simulink model "foot_placement_controller_in_simulink"  (R2019a)
settings: Solver=ode5  StartTime=0.0  StopTime=180  FixedStep=.005  RelTol=1e-3  EnableMultiTasking=on
undefined symbols (not defined in the file): CAN_Device, National_Instruments, PCI, Vector
libraries: dsparch4 x10, sldrtlib x5
settings Model: SimulationMode=external  ExtModeTrigDuration=60001  Creator=SD55648  LastModifiedBy=Huawei Wang
settings DataIOCC: LimitDataPoints=on  SaveFormat=Array  ReturnWorkspaceOutputs=off
settings OptimizationCC: LifeSpan=inf
settings DebuggingCC: SolverPrmCheckMsg=warning  SFUnexpectedBacktrackingDiag=warning  SFNoUnconditionalDefaultTransitionDiag=warning  SFExecutionAtInitializationDiag=none  ArithmeticOperatorsInVariantConditions=warning
settings HardwareCC: TargetBitPerLong=64  TargetBitPerPointer=64  TargetIntDivRoundTo=Zero  TargetEndianess=LittleEndian  TargetWordSize=64  TargetHWDeviceType=Intel->x86-64
settings ModelReferenceCC: PropagateSignalLabelsOutOfModel=off
settings SFSimCC: SimUseLocalCustomCode=off
settings RTWCC: SystemTargetFile=sldrt.tlc  TemplateMakefile=sldrt.tmf  Description=Simulink Desktop Real-Time  RTWUseLocalCustomCode=off  RTWCompilerOptimization=on
settings CodeAppCC: MaxIdLength=95  StateflowObjectComments=on
settings SimulinkDesktopRealTimeCC: TargetPreCompLibLocation=C:\Program Files\MATLAB\R2019a\toolbox\sldrt\lib\win64  TargetLangStandard=C89/C90 (ANSI)  SupportVariableSizeSignals=off  PreserveStateflowLocalDataDimensions=off
settings ConfigComp: CovMetricSettings=dw  CovHtmlReporting=on  CovSaveCumulativeToWorkspaceVar=on  CovSaveSingleToWorkspaceVar=on  CovExternalEMLEnable=off  CovSFcnEnable=off

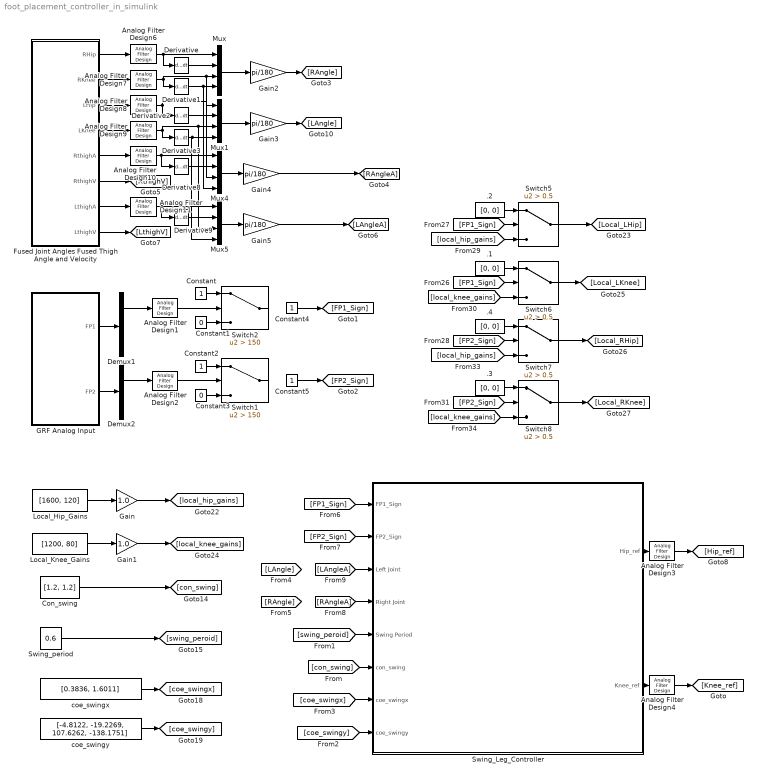
== system foot_placement_controller_in_simulink ==
  .{1..4} (4 alike) : Constant  Value=[0, 0]
  Analog Filter Design{1..4,6..11} (10 alike) : dsparch4/Analog Filter Design  method=Butterworth  filttype=Lowpass  N=2  Wlo=6*2*pi  Whi=80  Rp=2  Rs=40
  Con_swing : Constant  Value=[1.2, 1.2]
  Constant{,2,4..5} (4 alike) : Constant
  Constant1 : Constant  Value=0
  Constant3 : Constant  Value=0
  Demux1 : Demux  Outputs=6
  Demux2 : Demux  Outputs=6
  Derivative{,1..3,8..9} (6 alike) : Derivative
  Fused Joint Angles Fused Thigh Angle and Velocity : Subsystem
  "GRF Analog Input " : Subsystem
  Gain : Gain  Gain=1.0
  Gain1 : Gain  Gain=1.0
  Gain{2..5} (4 alike) : Gain  Gain=pi/180
  Local_Hip_Gains : Constant  Value=[1600, 120]
  Local_Knee_Gains : Constant  Value=[1200, 80]
  Mux{,1,4..5} (4 alike) : Mux
  "Swing_Leg_Controller " : Subsystem
  Swing_period : Constant  Value=0.6
  Switch1 : Switch  Criteria=u2 > Threshold  Threshold=150
  Switch2 : Switch  Criteria=u2 > Threshold  Threshold=150
  Switch{5..8} (4 alike) : Switch  Criteria=u2 > Threshold  Threshold=0.5
  coe_swingx : Constant  Value=[0.3836, 1.6011]
  coe_swingy : Constant  Value=[-4.8122, -19.2269, 107.6262, -138.1751]
  wires:
  Demux2/2 -> Analog Filter Design2/1
  "GRF Analog Input "/1(FP1) -> Demux1/1
  "GRF Analog Input "/2(FP2) -> Demux2/1
  Fused Joint Angles Fused Thigh Angle and Velocity/3(LHip) -> Analog Filter Design8/1
  Fused Joint Angles Fused Thigh Angle and Velocity/4(LKnee) -> Analog Filter Design9/1
  Fused Joint Angles Fused Thigh Angle and Velocity/5(RthighA) -> Analog Filter Design10/1
  Fused Joint Angles Fused Thigh Angle and Velocity/6(RthighV) -> [RthighV]
  Fused Joint Angles Fused Thigh Angle and Velocity/7(LthighA) -> Analog Filter Design11/1
  Fused Joint Angles Fused Thigh Angle and Velocity/8(LthighV) -> [LthighV]
  Derivative2/1 -> Mux1/2
  Derivative3/1 -> Mux1/4, Mux5/4
  Fused Joint Angles Fused Thigh Angle and Velocity/1(RHip) -> Analog Filter Design6/1
  Derivative/1 -> Mux/2
  Fused Joint Angles Fused Thigh Angle and Velocity/2(RKnee) -> Analog Filter Design7/1
  Derivative1/1 -> Mux4/4, Mux/4
  Mux1/1 -> Gain3/1
  Demux1/2 -> Analog Filter Design1/1
  Constant/1 -> Switch2/1
  Constant1/1 -> Switch2/3
  Constant2/1 -> Switch1/1
  Constant3/1 -> Switch1/3
  Mux/1 -> Gain2/1
  Gain3/1 -> [LAngle]
  Gain2/1 -> [RAngle]
  Con_swing/1 -> [con_swing]
  Swing_period/1 -> [swing_peroid]
  coe_swingx/1 -> [coe_swingx]
  [FP1_Sign] -> Switch5/2
  Local_Hip_Gains/1 -> Gain/1
  Local_Knee_Gains/1 -> Gain1/1
  [local_hip_gains] -> Switch5/3
  .2/1 -> Switch5/1
  [FP1_Sign] -> Switch6/2
  [local_knee_gains] -> Switch6/3
  .1/1 -> Switch6/1
  [FP2_Sign] -> Switch7/2
  [local_hip_gains] -> Switch7/3
  .4/1 -> Switch7/1
  [FP2_Sign] -> Switch8/2
  [local_knee_gains] -> Switch8/3
  .3/1 -> Switch8/1
  Switch5/1 -> [Local_LHip]
  Switch6/1 -> [Local_LKnee]
  Switch7/1 -> [Local_RHip]
  Switch8/1 -> [Local_RKnee]
  coe_swingy/1 -> [coe_swingy]
  [con_swing] -> "Swing_Leg_Controller "/6(con_swing)
  [swing_peroid] -> "Swing_Leg_Controller "/5(Swing Period)
  [coe_swingy] -> "Swing_Leg_Controller "/8(coe_swingy)
  [coe_swingx] -> "Swing_Leg_Controller "/7(coe_swingx)
  [LAngleA] -> "Swing_Leg_Controller "/3(Left Joint)
  [RAngleA] -> "Swing_Leg_Controller "/4(Right Joint)
  [FP1_Sign] -> "Swing_Leg_Controller "/1(FP1_Sign)
  [FP2_Sign] -> "Swing_Leg_Controller "/2(FP2_Sign)
  Gain/1 -> [local_hip_gains]
  Gain1/1 -> [local_knee_gains]
  Analog Filter Design6/1 -> Mux/1, Derivative/1
  Analog Filter Design7/1 -> Derivative1/1, Mux4/3, Mux/3
  Analog Filter Design8/1 -> Mux1/1, Derivative2/1
  Analog Filter Design9/1 -> Derivative3/1, Mux1/3, Mux5/3
  Analog Filter Design10/1 -> Mux4/1, Derivative8/1
  Analog Filter Design11/1 -> Derivative9/1, Mux5/1
  Derivative8/1 -> Mux4/2
  Mux4/1 -> Gain4/1
  Derivative9/1 -> Mux5/2
  Gain5/1 -> [LAngleA]
  Mux5/1 -> Gain5/1
  Gain4/1 -> [RAngleA]
  Analog Filter Design1/1 -> Switch2/2
  Analog Filter Design2/1 -> Switch1/2
  "Swing_Leg_Controller "/2(Knee_ref) -> Analog Filter Design4/1
  "Swing_Leg_Controller "/1("Hip_ref ") -> Analog Filter Design3/1
  Analog Filter Design3/1 -> [Hip_ref]
  Analog Filter Design4/1 -> [Knee_ref]
  Constant4/1 -> [FP1_Sign]
  Constant5/1 -> [FP2_Sign]

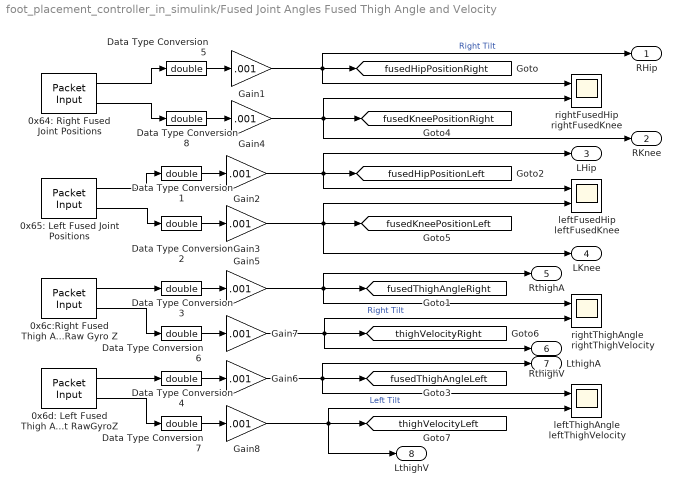
== system foot_placement_controller_in_simulink/Fused Joint Angles Fused Thigh Angle and Velocity ==
  0x64: Right Fused Joint Positions : sldrtlib/Packet Input  SampleTime=.005  MaxMissedTicks=10  ShowMissedTicks=off  YieldWhenWaiting=off  DrvName=Vector/CAN_Device  DrvAddress=1  DrvOptions=[0 0 0 0 1000]  PacketSize=8  DataTypes={'int32','int32'}  ShowReady=off  ShowError=off  PacketID=2048e0 + (hex2dec('64'))  ByteOrder=1  ShowTimestamp=off
      settings: AttributesFormatString=Vector\nCAN Device [1h]  SourceProductName=Simulink Desktop Real-Time
  0x65: Left Fused Joint Positions : sldrtlib/Packet Input  SampleTime=.005  MaxMissedTicks=10  ShowMissedTicks=off  YieldWhenWaiting=off  DrvName=Vector/CAN_Device  DrvAddress=1  DrvOptions=[0 0 0 0 1000]  PacketSize=8  DataTypes={'int32','int32'}  ShowReady=off  ShowError=off  PacketID=2048e0 + (hex2dec('65'))  ByteOrder=1  ShowTimestamp=off
      settings: AttributesFormatString=Vector\nCAN Device [1h]  SourceProductName=Simulink Desktop Real-Time
  0x6c:Right Fused Thigh Angle/Tilt Raw Gyro Z : sldrtlib/Packet Input  SampleTime=.005  MaxMissedTicks=10  ShowMissedTicks=off  YieldWhenWaiting=off  DrvName=Vector/CAN_Device  DrvAddress=1  DrvOptions=[0 0 0 0 1000]  PacketSize=8  DataTypes={'int32','int32'}  ShowReady=off  ShowError=off  PacketID=2048e0 + (hex2dec('6c'))  ByteOrder=1  ShowTimestamp=off
      settings: AttributesFormatString=Vector\nCAN Device [1h]  SourceProductName=Simulink Desktop Real-Time
  0x6d: Left Fused Thigh Angle/Tilt RawGyroZ : sldrtlib/Packet Input  SampleTime=.005  MaxMissedTicks=10  ShowMissedTicks=off  YieldWhenWaiting=off  DrvName=Vector/CAN_Device  DrvAddress=1  DrvOptions=[0 0 0 0 1000]  PacketSize=8  DataTypes={'int32','int32'}  ShowReady=off  ShowError=off  PacketID=2048e0 + (hex2dec('6d'))  ByteOrder=1  ShowTimestamp=off
      settings: AttributesFormatString=Vector\nCAN Device [1h]  SourceProductName=Simulink Desktop Real-Time
  Data Type Conversion{1..8} (8 alike) : DataTypeConversion  OutDataTypeStr=double
  Gain{1..8} (8 alike) : Gain  Gain=.001
  leftFusedHip leftFusedKnee : Scope  NumInputPorts=2
  leftThighAngle leftThighVelocity : Scope  NumInputPorts=2
  rightFusedHip rightFusedKnee : Scope  NumInputPorts=2
  rightThighAngle rightThighVelocity : Scope  NumInputPorts=2
  RHip : Outport
  RKnee : Outport  Port=2
  LHip : Outport  Port=3
  LKnee : Outport  Port=4
  RthighA : Outport  Port=5
  RthighV : Outport  Port=6
  LthighA : Outport  Port=7
  LthighV : Outport  Port=8
  tag scope: fusedHipPositionLeft=global, fusedHipPositionRight=global, fusedKneePositionLeft=global, fusedKneePositionRight=global, fusedThighAngleLeft=global, fusedThighAngleRight=global, thighVelocityLeft=global, thighVelocityRight=global
  wires:
  Gain8/1 -> LthighV/1, [thighVelocityLeft], leftThighAngle leftThighVelocity/2
  Gain7/1 -> RthighV/1, [thighVelocityRight], rightThighAngle rightThighVelocity/2
  0x6d: Left Fused Thigh Angle/Tilt RawGyroZ/2 -> Data Type Conversion7/1
  0x6c:Right Fused Thigh Angle/Tilt Raw Gyro Z/2 -> Data Type Conversion6/1
  Data Type Conversion7/1 -> Gain8/1
  Data Type Conversion6/1 -> Gain7/1
  Gain6/1 -> leftThighAngle leftThighVelocity/1, LthighA/1, [fusedThighAngleLeft]  "Left Tilt"
  Gain5/1 -> RthighA/1, [fusedThighAngleRight], rightThighAngle rightThighVelocity/1  "Right Tilt"
  Gain3/1 -> LKnee/1, [fusedKneePositionLeft], leftFusedHip leftFusedKnee/2
  Gain2/1 -> LHip/1, [fusedHipPositionLeft], leftFusedHip leftFusedKnee/1
  Gain4/1 -> RKnee/1, [fusedKneePositionRight], rightFusedHip rightFusedKnee/2
  Gain1/1 -> RHip/1, [fusedHipPositionRight], rightFusedHip rightFusedKnee/1  "Right Tilt"
  Data Type Conversion4/1 -> Gain6/1
  Data Type Conversion3/1 -> Gain5/1
  Data Type Conversion2/1 -> Gain3/1
  Data Type Conversion1/1 -> Gain2/1
  Data Type Conversion8/1 -> Gain4/1
  Data Type Conversion5/1 -> Gain1/1
  0x65: Left Fused Joint Positions/2 -> Data Type Conversion2/1
  0x65: Left Fused Joint Positions/1 -> Data Type Conversion1/1
  0x64: Right Fused Joint Positions/2 -> Data Type Conversion8/1
  0x64: Right Fused Joint Positions/1 -> Data Type Conversion5/1
  0x6d: Left Fused Thigh Angle/Tilt RawGyroZ/1 -> Data Type Conversion4/1
  0x6c:Right Fused Thigh Angle/Tilt Raw Gyro Z/1 -> Data Type Conversion3/1

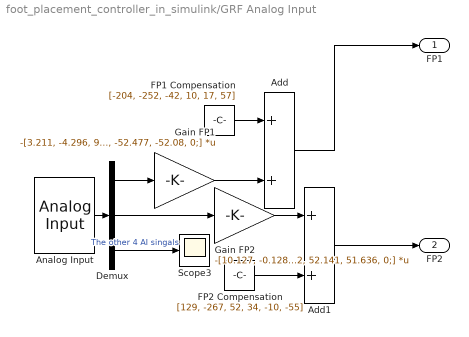
== system foot_placement_controller_in_simulink/GRF Analog Input  ==
  Add : Sum
  Add1 : Sum
  Analog Input : sldrtlib/Analog Input  SampleTime=0.005  MaxMissedTicks=100  ShowMissedTicks=off  YieldWhenWaiting=off  DrvName=National_Instruments/PCI-6014  DrvAddress=4294967295  DrvOptions=[2 0 0 0 0 0]  Channels=[1:16]  RangeMode=1  VoltRange=1  DataType=1
      settings: AttributesFormatString=National Instruments\nPCI-6014 [auto]  SourceProductName=Simulink Desktop Real-Time
  Demux : Demux  Outputs=3
  FP1 Compensation : Constant  Value=[-204, -252, -42, 10, 17, 57]
  FP2 Compensation : Constant  Value=[129, -267, 52, 34, -10, -55]
  Gain FP1 : Gain  Gain=-[3.211, -4.296, 9.517, -506.156, -503.077, -12.798; -488.7, -489.177, -490.137, 12.72, -12.405, 6.997; -2.439, -22.137, -12.713, -5.808, 0.306, -529.752; 51.205, -296.238, 301.239, 0, 0, 54.628; 0, 0, 0, -252.497, 357.263, -9.06; 249.758, 24.2, 20.303, -52.477, -52.08, 0;]  Multiplication=Matrix(K*u) (u vector)
  "Gain FP2 " : Gain  Gain=-[10.127, -0.128, 7.117, 502.928, 498.685, -10.051; -485.724, -486.699, -488.278, 16.96, 24.012, 1.989; -3.781, -5.618, -17.688, -4.968, 0.7, -516.168; 297.882, -297.409, 45.867, 0, 0, 52.865; 0, 0, 0, -357.685, 248.453, 8.76; -30.947, -27.516, -254.202, 52.141, 51.636, 0;]  Multiplication=Matrix(K*u) (u vector)
  Scope3 : Scope
  FP1 : Outport
  FP2 : Outport  Port=2
  wires:
  Demux/3 -> Scope3/1  "The other 4 AI singals"
  Demux/1 -> Gain FP1/1
  Analog Input/1 -> Demux/1
  Gain FP1/1 -> Add/2
  FP1 Compensation/1 -> Add/1
  "Gain FP2 "/1 -> Add1/1
  FP2 Compensation/1 -> Add1/2
  Demux/2 -> "Gain FP2 "/1
  Add1/1 -> FP2/1
  Add/1 -> FP1/1

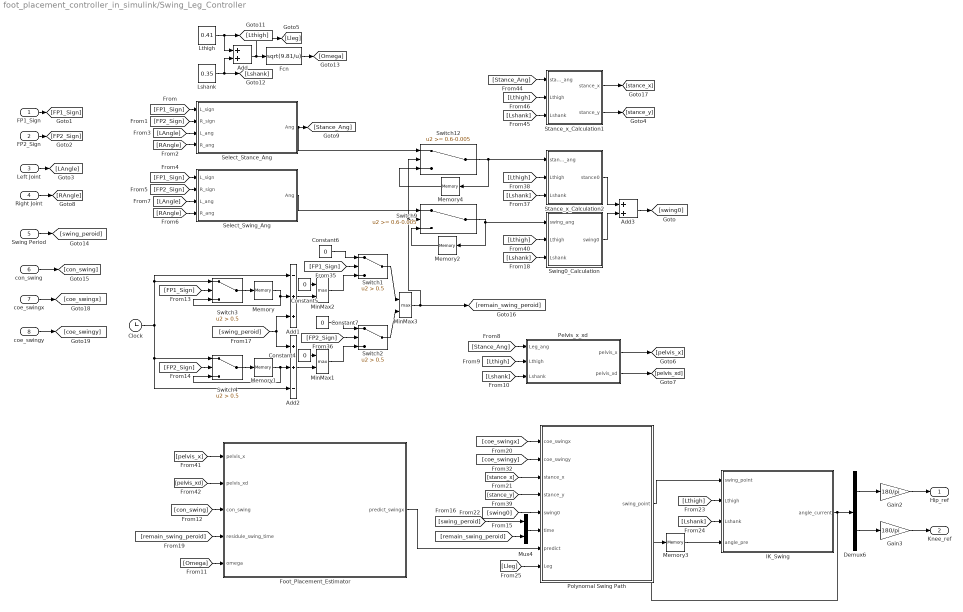
== system foot_placement_controller_in_simulink/Swing_Leg_Controller  ==
  FP1_Sign : Inport
  FP2_Sign : Inport  Port=2
  Left Joint : Inport  Port=3
  Right Joint : Inport  Port=4
  Swing Period : Inport  Port=5
  con_swing : Inport  Port=6
  coe_swingx : Inport  Port=7
  coe_swingy : Inport  Port=8
  Add : Sum
  Add1 : Sum  Inputs=-++
  Add2 : Sum  Inputs=++-
  Add3 : Sum
  Clock : Clock
  Constant{4..7} (4 alike) : Constant  Value=0
  Demux6 : Demux  Outputs=2
  Fcn : Fcn  Expr=sqrt(9.81/u)
  Foot_Placement_Estimator : MATLAB Function  TreatAsAtomicUnit=on
  Gain2 : Gain  Gain=180/pi
  Gain3 : Gain  Gain=180/pi
  IK_Swing : MATLAB Function  TreatAsAtomicUnit=on
  Lshank : Constant  Value=0.35
  Lthigh : Constant  Value=0.41
  Memory{,1..2,4} (4 alike) : Memory
  Memory3 : Memory  InitialCondition=[-pi/9, pi/18]
  MinMax1 : MinMax  Function=max  Inputs=2
  MinMax2 : MinMax  Function=max  Inputs=2
  MinMax3 : MinMax  Function=max  Inputs=2
  Mux4 : Mux  Inputs=2
  Pelvis_x_xd : MATLAB Function  TreatAsAtomicUnit=on
  Polynomal Swing Path : MATLAB Function  TreatAsAtomicUnit=on
  Select_Stance_Ang : MATLAB Function  TreatAsAtomicUnit=on
  Select_Swing_Ang : MATLAB Function  TreatAsAtomicUnit=on
  Stance_x_Calculation1 : MATLAB Function  TreatAsAtomicUnit=on
  Stance_x_Calculation2 : MATLAB Function  TreatAsAtomicUnit=on
  Swing0_Calculation : MATLAB Function  TreatAsAtomicUnit=on
  Switch{1..4} (4 alike) : Switch  Criteria=u2 > Threshold  Threshold=0.5
  Switch12 : Switch  Threshold=0.6-0.005
  Switch9 : Switch  Threshold=0.6-0.005
  "Hip_ref " : Outport
  Knee_ref : Outport  Port=2
  wires:
  [stance_x] -> Polynomal Swing Path/3(stance_x)
  Pelvis_x_xd/1(pelvis_x) -> [pelvis_x]
  Foot_Placement_Estimator/1(predict_swingx) -> Polynomal Swing Path/7(predict)
  Pelvis_x_xd/2(pelvis_xd) -> [pelvis_xd]
  Lthigh/1 -> [Lthigh], Add/1
  [remain_swing_peroid] -> Mux4/2
  [swing_peroid] -> Mux4/1
  [remain_swing_peroid] -> Foot_Placement_Estimator/4(residule_swing_time)
  [FP1_Sign] -> Switch3/2
  Clock/1 -> Add1/1, Switch3/1, Add2/3, Switch4/1
  Polynomal Swing Path/1(swing_point) -> IK_Swing/1(swing_point)
  [Stance_Ang] -> Pelvis_x_xd/1(Leg_ang)
  [Omega] -> Foot_Placement_Estimator/5(omega)
  [RAngle] -> Select_Swing_Ang/4(R_ang)
  Switch3/1 -> Memory/1
  Fcn/1 -> [Omega]
  Select_Swing_Ang/1(Ang) -> Switch9/1
  [Lthigh] -> Pelvis_x_xd/2(Lthigh)
  [Lshank] -> Pelvis_x_xd/3(Lshank)
  [FP2_Sign] -> Switch4/2
  Switch4/1 -> Memory1/1
  Lshank/1 -> Add/2, [Lshank]
  Add/1 -> [Lleg], Fcn/1
  [FP2_Sign] -> Select_Stance_Ang/2(R_sign)
  Select_Stance_Ang/1(Ang) -> Switch12/1, [Stance_Ang]
  [LAngle] -> Select_Stance_Ang/3(L_ang)
  [con_swing] -> Foot_Placement_Estimator/3(con_swing)
  [RAngle] -> Select_Stance_Ang/4(R_ang)
  [LAngle] -> Select_Swing_Ang/3(L_ang)
  Memory/1 -> Add1/2, Switch3/3
  Memory1/1 -> Add2/2, Switch4/3
  [FP1_Sign] -> Select_Stance_Ang/1(L_sign)
  [FP2_Sign] -> Select_Swing_Ang/2(R_sign)
  [FP1_Sign] -> Select_Swing_Ang/1(L_sign)
  [Lshank] -> IK_Swing/3(Lshank)
  Demux6/1 -> Gain2/1
  IK_Swing/1(angle_current) -> Memory3/1, Demux6/1
  [swing0] -> Polynomal Swing Path/5(swing0)
  Demux6/2 -> Gain3/1
  Mux4/1 -> Polynomal Swing Path/6(time)
  [coe_swingx] -> Polynomal Swing Path/1(coe_swingx)
  [Lthigh] -> IK_Swing/2(Lthigh)
  Memory3/1 -> IK_Swing/4(angle_pre)
  MinMax2/1 -> Switch1/3
  Constant5/1 -> MinMax2/1
  [Lthigh] -> Swing0_Calculation/2(Lthigh)
  [Lshank] -> Swing0_Calculation/3(Lshank)
  Constant4/1 -> MinMax1/1
  [swing_peroid] -> Add1/3, Add2/1
  MinMax3/1 -> Switch12/2, Switch9/2, [remain_swing_peroid]
  Add2/1 -> MinMax1/2
  Switch2/1 -> MinMax3/2
  Memory2/1 -> Switch9/3
  [FP1_Sign] -> Switch1/2
  Constant6/1 -> Switch1/1
  [FP2_Sign] -> Switch2/2
  Add1/1 -> MinMax2/2
  MinMax1/1 -> Switch2/3
  Constant7/1 -> Switch2/1
  Switch1/1 -> MinMax3/1
  Switch9/1 -> Memory2/1, Swing0_Calculation/1(swing_ang)
  Swing0_Calculation/1(swing0) -> Add3/2
  [Lthigh] -> Stance_x_Calculation1/2(Lthigh)
  Stance_x_Calculation1/1(stance_x) -> [stance_x]
  [pelvis_x] -> Foot_Placement_Estimator/1(pelvis_x)
  [Lshank] -> Stance_x_Calculation1/3(Lshank)
  [Stance_Ang] -> Stance_x_Calculation1/1(stance_ang)
  [pelvis_xd] -> Foot_Placement_Estimator/2(pelvis_xd)
  [stance_y] -> Polynomal Swing Path/4(stance_y)
  [Lshank] -> Stance_x_Calculation2/3(Lshank)
  Stance_x_Calculation2/1(stance0) -> Add3/1
  Switch12/1 -> Stance_x_Calculation2/1(stance_ang), Memory4/1
  [Lthigh] -> Stance_x_Calculation2/2(Lthigh)
  Memory4/1 -> Switch12/3
  [coe_swingy] -> Polynomal Swing Path/2(coe_swingy)
  Add3/1 -> [swing0]
  Stance_x_Calculation1/2(stance_y) -> [stance_y]
  [Lleg] -> Polynomal Swing Path/8(Leg)
  FP1_Sign/1 -> [FP1_Sign]
  FP2_Sign/1 -> [FP2_Sign]
  Left Joint/1 -> [LAngle]
  Right Joint/1 -> [RAngle]
  Swing Period/1 -> [swing_peroid]
  con_swing/1 -> [con_swing]
  coe_swingx/1 -> [coe_swingx]
  coe_swingy/1 -> [coe_swingy]
  Gain2/1 -> "Hip_ref "/1
  Gain3/1 -> Knee_ref/1

== matlab function foot_placement_controller_in_simulink/Swing_Leg_Controller /Foot_Placement_Estimator ==
  data: pelvis_x input; predict_swingx output; pelvis_xd input; con_swing input; residule_swing_time input; omega input
function predict_swingx = foot_placement_estimation(pelvis_x, pelvis_xd,...
                        con_swing, residule_swing_time, omega)
  
    predict_swingx0 = con_swing(1)*pelvis_x + con_swing(2)*pelvis_xd/omega;
    
    predict_swingx = (predict_swingx0)*exp(omega*1*residule_swing_time);

end

== matlab function foot_placement_controller_in_simulink/Swing_Leg_Controller /Pelvis_x_xd ==
  data: Leg_ang input; pelvis_x output; Lthigh input; Lshank input; pelvis_xd output
function [pelvis_x, pelvis_xd] = plevis_state(Leg_ang, Lthigh, Lshank)
    
    pelvis_x = -Lthigh*sin(Leg_ang(1))... 
               -Lshank*sin(Leg_ang(1) - Leg_ang(3));
        
    pelvis_xd = -Lthigh*cos(Leg_ang(1))*Leg_ang(2)...
                -Lshank*cos(Leg_ang(1) - Leg_ang(3))*(Leg_ang(2) - Leg_ang(4));
    
end

== matlab function foot_placement_controller_in_simulink/Swing_Leg_Controller /Polynomal Swing Path ==
  data: coe_swingx input; coe_swingy input; stance_x input; stance_y input; swing_point output; swing0 input; time input; predict input; Leg input
function swing_point = swing_current_point(coe_swingx, coe_swingy, stance_x,...
                    stance_y, swing0, time, predict, Leg)
         
    swing_tp = time(1);
    swing_t = time(1) - time(2);
     
    B = coe_swingx(1);
    C = coe_swingx(2);
    
    By = coe_swingy(1);
    Cy = coe_swingy(2);
    Dy = coe_swingy(3);
    Ey = coe_swingy(4);
    
    
    Scale = predict - swing0(1);
    
    Scale_y = 0.03 - swing0(2);
    
    ScaleT = (swing_t)/(swing_tp);

    swing_x = (swing0(1) + B*Scale*ScaleT + C*Scale*ScaleT^2 ... 
                 + (1 - B - C)*Scale*ScaleT^3) - stance_x; 
             
    swing_y = (swing0(2) + By*Scale_y*ScaleT + Cy*Scale_y*ScaleT^2 ... 
                 + Dy*Scale_y*ScaleT^3 + Ey*Scale_y*ScaleT^4 ...
                 + (1 - By - Cy - Dy - Ey)*Scale_y*ScaleT^5) - stance_y; 
             
    swing_point = [swing_x, swing_y];
end

== matlab function foot_placement_controller_in_simulink/Swing_Leg_Controller /IK_Swing ==
  data: swing_point input; angle_current output; Lthigh input; Lshank input; angle_pre input
function angle_current = IK_swing(swing_point, Lthigh, Lshank, angle_pre)

    x = [angle_pre(1), angle_pre(2)]';

    Lleg = Lthigh + Lshank;

    if sqrt(swing_point(1)^2 + swing_point(2)^2) > Lleg
        swing_point(2) = -sqrt(Lleg^2 - swing_point(1)^2);
    end
    
    for i = 1:50

        f = zeros(2, 1);

        f(1) = Lthigh*sin(x(1)) + Lshank*sin(x(1) - x(2)) - swing_point(1); 
        f(2) = -Lthigh*cos(x(1)) - Lshank*cos(x(1) - x(2)) - swing_point(2);


        dfdx = zeros(2, 2);

        dfdx(1, 1) = Lthigh*cos(x(1)) + Lshank*cos(x(1) - x(2));
        dfdx(1, 2) = -Lshank*cos(x(1) - x(2));

        dfdx(2, 1) = Lthigh*sin(x(1)) + Lshank*sin(x(1) - x(2));
        dfdx(2, 2) = -Lshank*sin(x(1) - x(2));

        x = x - dfdx\f;

        if x(1) <= -pi/8
            x(1) = -pi/8;
        elseif x(1) >= pi/2.1
            x(1) = pi/2.1;
        end

        if x(2) <= 0
            x(2) = 0;
        elseif x(2) >= pi/2
            x(2) = pi/2;
        end

        
        if max(abs(f)) < 1e-4
            break;
        end
    end
    
    angle_current = x;
end

== matlab function foot_placement_controller_in_simulink/Swing_Leg_Controller /Select_Stance_Ang ==
  data: L_sign input; Ang output; R_sign input; L_ang input; R_ang input
function Ang = Ang_Stance_Select(L_sign, R_sign, L_ang, R_ang)

if L_sign == 0
    Ang = R_ang;
elseif R_sign == 0
    Ang = L_ang;
else
    Ang = [0, 0, 0, 0]';
end

end

== matlab function foot_placement_controller_in_simulink/Swing_Leg_Controller /Select_Swing_Ang ==
  data: L_sign input; Ang output; R_sign input; L_ang input; R_ang input
function Ang = Ang_Swing_Select(L_sign, R_sign, L_ang, R_ang)

if L_sign == 0
    Ang = L_ang;
elseif R_sign == 0
    Ang = R_ang;
else
    Ang = [0, 0, 0, 0]';
end

end

== matlab function foot_placement_controller_in_simulink/Swing_Leg_Controller /Stance_x_Calculation2 ==
  data: stance_ang input; stance0 output; Lthigh input; Lshank input
function stance0 = fcn(stance_ang, Lthigh, Lshank)

hip_ang = stance_ang(1);
knee_ang = stance_ang(3);

stance_x = -Lthigh*sin(hip_ang) - Lshank*sin(hip_ang - knee_ang);
stance_y =  Lthigh*cos(hip_ang) + Lshank*cos(hip_ang - knee_ang);

stance0 = [stance_x, stance_y];

end

== matlab function foot_placement_controller_in_simulink/Swing_Leg_Controller /Swing0_Calculation ==
  data: swing_ang input; swing0 output; Lthigh input; Lshank input
function swing0 = swing0_cal(swing_ang, Lthigh, Lshank)

hip_ang = swing_ang(1);
knee_ang = swing_ang(3);

swing_x = Lthigh*sin(hip_ang) + Lshank*sin(hip_ang - knee_ang);

swing_y = -Lthigh*cos(hip_ang) - Lshank*cos(hip_ang - knee_ang);

swing0 = [swing_x, swing_y];

end

== matlab function foot_placement_controller_in_simulink/Swing_Leg_Controller /Stance_x_Calculation1 ==
  data: stance_ang input; stance_x output; Lthigh input; Lshank input; stance_y output
function [stance_x, stance_y] = fcn(stance_ang, Lthigh, Lshank)

hip_ang = stance_ang(1);
knee_ang = stance_ang(3);

stance_x = -Lthigh*sin(hip_ang) - Lshank*sin(hip_ang - knee_ang);

stance_y = Lthigh*cos(hip_ang) + Lshank*cos(hip_ang - knee_ang);

end
